simulink model "nuclearReactor"  (R2014b)
settings: Solver=ode1  StartTime=0.0  StopTime=100  FixedStep=0.0001  MaxStep=0.0001  RelTol=1e-3
(part 1 of 4)
settings Model: Creator=sand080  LastModifiedBy=nall426
settings DataIOCC: LimitDataPoints=off
settings RTWCC: CustomInitializer=gettimeofday(&t0, 0);
settings RTWCC: CustomSourceCode=|
  | int gettimeofday(struct timeval * tp, struct timezone * tzp)
  | {
  |     // Note: some broken versions only have 8 trailing zero's, the correct epoch has 9 trailing zero's
  |     static const uint64_t EPOCH = ((uint64_t) 116444736000000000ULL);
  | 
  |     SYSTEMTIME  system_time;
  |     FILETIME    file_time;
  |     uint64_t    time;
  | 
  | 	GetSystemTime( &system_time );
  |     SystemTimeToFileTime( &system_time, &file_time );
  |     time =  ((uint64_t)file_time.dwLowDateTime )      ;
  |     time += ((uint64_t)file_time.dwHighDateTime) << 32;
  | 
  |     tp->tv_sec  = (long) ((time - EPOCH) / 10000000L);
  |     tp->tv_usec = (long) (system_time.wMilliseconds * 1000);
  |     return 0;
  | }
  | 
  | struct timeval t0, t1;
settings RTWCC: CustomHeaderCode=|
  | #include <stdint.h> // portable: uint64_t   MSVC: __int64
  | #include <Windows.h>
settings RTWCC: CustomTerminator=|
  | gettimeofday(&t1, 0);
  | 
  | long elapsed = (t1.tv_sec-t0.tv_sec)*1000000 + t1.tv_usec-t0.tv_usec;
  | printf("Time taken: %ld microseconds (%.3f seconds)\n", elapsed, (elapsed / 1000000.0));

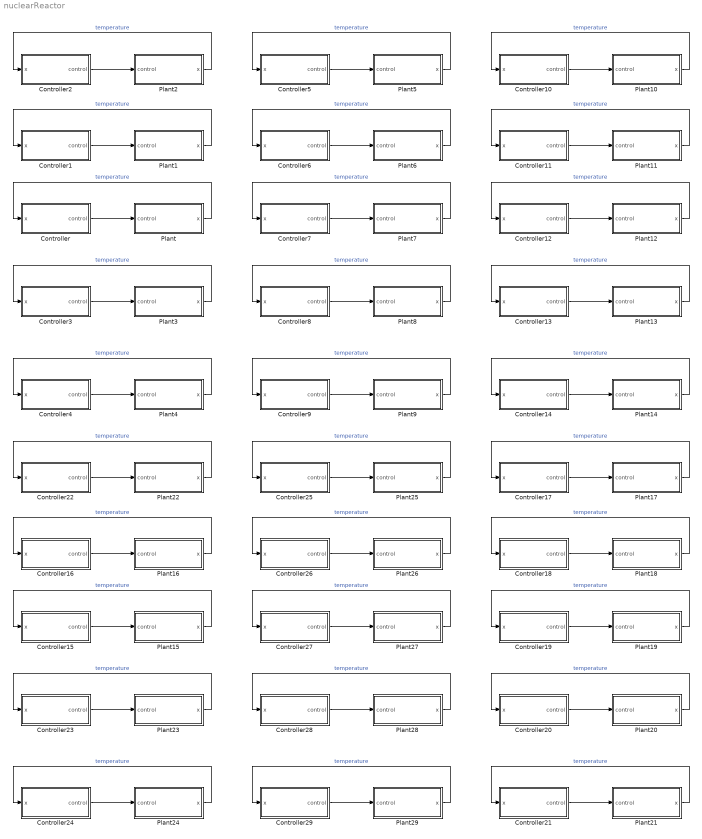
== system nuclearReactor ==
  Controller : Subsystem
  Controller1 : Subsystem
  Controller10 : Subsystem
  Controller11 : Subsystem
  Controller12 : Subsystem
  Controller13 : Subsystem
  Controller14 : Subsystem
  Controller15 : Subsystem
  Controller16 : Subsystem
  Controller17 : Subsystem
  Controller18 : Subsystem
  Controller19 : Subsystem
  Controller2 : Subsystem
  Controller20 : Subsystem
  Controller21 : Subsystem
  Controller22 : Subsystem
  Controller23 : Subsystem
  Controller24 : Subsystem
  Controller25 : Subsystem
  Controller26 : Subsystem
  Controller27 : Subsystem
  Controller28 : Subsystem
  Controller29 : Subsystem
  Controller3 : Subsystem
  Controller4 : Subsystem
  Controller5 : Subsystem
  Controller6 : Subsystem
  Controller7 : Subsystem
  Controller8 : Subsystem
  Controller9 : Subsystem
  Plant : Subsystem
  Plant1 : Subsystem
  Plant10 : Subsystem
  Plant11 : Subsystem
  Plant12 : Subsystem
  Plant13 : Subsystem
  Plant14 : Subsystem
  Plant15 : Subsystem
  Plant16 : Subsystem
  Plant17 : Subsystem
  Plant18 : Subsystem
  Plant19 : Subsystem
  Plant2 : Subsystem
  Plant20 : Subsystem
  Plant21 : Subsystem
  Plant22 : Subsystem
  Plant23 : Subsystem
  Plant24 : Subsystem
  Plant25 : Subsystem
  Plant26 : Subsystem
  Plant27 : Subsystem
  Plant28 : Subsystem
  Plant29 : Subsystem
  Plant3 : Subsystem
  Plant4 : Subsystem
  Plant5 : Subsystem
  Plant6 : Subsystem
  Plant7 : Subsystem
  Plant8 : Subsystem
  Plant9 : Subsystem
  wires:
  Controller/1(control) -> Plant/1(control)
  Plant/1(x) -> Controller/1(x)  "temperature"
  Controller1/1(control) -> Plant1/1(control)
  Plant1/1(x) -> Controller1/1(x)  "temperature"
  Controller2/1(control) -> Plant2/1(control)
  Plant2/1(x) -> Controller2/1(x)  "temperature"
  Controller3/1(control) -> Plant3/1(control)
  Plant3/1(x) -> Controller3/1(x)  "temperature"
  Controller4/1(control) -> Plant4/1(control)
  Plant4/1(x) -> Controller4/1(x)  "temperature"
  Controller5/1(control) -> Plant5/1(control)
  Plant5/1(x) -> Controller5/1(x)  "temperature"
  Controller6/1(control) -> Plant6/1(control)
  Plant6/1(x) -> Controller6/1(x)  "temperature"
  Controller7/1(control) -> Plant7/1(control)
  Plant7/1(x) -> Controller7/1(x)  "temperature"
  Controller8/1(control) -> Plant8/1(control)
  Plant8/1(x) -> Controller8/1(x)  "temperature"
  Controller9/1(control) -> Plant9/1(control)
  Plant9/1(x) -> Controller9/1(x)  "temperature"
  Controller10/1(control) -> Plant10/1(control)
  Plant10/1(x) -> Controller10/1(x)  "temperature"
  Controller11/1(control) -> Plant11/1(control)
  Plant11/1(x) -> Controller11/1(x)  "temperature"
  Controller12/1(control) -> Plant12/1(control)
  Plant12/1(x) -> Controller12/1(x)  "temperature"
  Controller13/1(control) -> Plant13/1(control)
  Plant13/1(x) -> Controller13/1(x)  "temperature"
  Controller14/1(control) -> Plant14/1(control)
  Plant14/1(x) -> Controller14/1(x)  "temperature"
  Controller15/1(control) -> Plant15/1(control)
  Plant15/1(x) -> Controller15/1(x)  "temperature"
  Controller16/1(control) -> Plant16/1(control)
  Plant16/1(x) -> Controller16/1(x)  "temperature"
  Controller22/1(control) -> Plant22/1(control)
  Plant22/1(x) -> Controller22/1(x)  "temperature"
  Controller23/1(control) -> Plant23/1(control)
  Plant23/1(x) -> Controller23/1(x)  "temperature"
  Controller24/1(control) -> Plant24/1(control)
  Plant24/1(x) -> Controller24/1(x)  "temperature"
  Controller25/1(control) -> Plant25/1(control)
  Plant25/1(x) -> Controller25/1(x)  "temperature"
  Controller26/1(control) -> Plant26/1(control)
  Plant26/1(x) -> Controller26/1(x)  "temperature"
  Controller27/1(control) -> Plant27/1(control)
  Plant27/1(x) -> Controller27/1(x)  "temperature"
  Controller28/1(control) -> Plant28/1(control)
  Plant28/1(x) -> Controller28/1(x)  "temperature"
  Controller29/1(control) -> Plant29/1(control)
  Plant29/1(x) -> Controller29/1(x)  "temperature"
  Controller17/1(control) -> Plant17/1(control)
  Plant17/1(x) -> Controller17/1(x)  "temperature"
  Controller18/1(control) -> Plant18/1(control)
  Plant18/1(x) -> Controller18/1(x)  "temperature"
  Controller19/1(control) -> Plant19/1(control)
  Plant19/1(x) -> Controller19/1(x)  "temperature"
  Controller20/1(control) -> Plant20/1(control)
  Plant20/1(x) -> Controller20/1(x)  "temperature"
  Controller21/1(control) -> Plant21/1(control)
  Plant21/1(x) -> Controller21/1(x)  "temperature"

== system nuclearReactor/Controller ==
  x : Inport
  INIT y1 : Constant  Value=0
  INIT y2 : Constant  Value=0
  Integrator t1 : DiscreteIntegrator  ExternalReset=either  InitialConditionSource=external  InitialCondition=510  InitialConditionSetting=State (most efficient)  SampleTime=-1
  Integrator t2 : DiscreteIntegrator  ExternalReset=either  InitialConditionSource=external  InitialCondition=510  InitialConditionSetting=State (most efficient)  SampleTime=-1
  MATLAB Function : MATLAB Function  Priority=1  TreatAsAtomicUnit=on
  Scope : Scope  NumInputPorts=8
      settings: TickLabels=on  ShowLegends=on  YMin=0~0~0~0~0~0~0~0  YMax=1~1~1~1~1~1~1~1
  con1 : Constant
  con2 : Constant
  q : Memory  LinearizeMemory=on
  reset1 : Memory  LinearizeMemory=on
  reset2 : Memory  LinearizeMemory=on
  control : Outport
  wires:
  MATLAB Function/4(control) -> Scope/1, control/1  "control"
  INIT y1/1 -> Integrator t1/3
  INIT y2/1 -> Integrator t2/3
  con1/1 -> Integrator t1/1
  MATLAB Function/1(qNext) -> q/1  "q_before"
  q/1 -> MATLAB Function/1(q)  "q_after"
  MATLAB Function/2(r1) -> reset1/1
  reset1/1 -> Integrator t1/2  "reset_after"
  x/1 -> Scope/8, MATLAB Function/2(x)
  con2/1 -> Integrator t2/1
  Integrator t1/1 -> MATLAB Function/3(y1), Scope/2  "integrator t1"
  Integrator t2/1 -> MATLAB Function/4(y2), Scope/3  "integrator t2"
  reset2/1 -> Integrator t2/2
  MATLAB Function/3(r2) -> reset2/1

== system nuclearReactor/Controller1 ==
  x : Inport
  INIT y1 : Constant  Value=0
  INIT y2 : Constant  Value=0
  Integrator t1 : DiscreteIntegrator  ExternalReset=either  InitialConditionSource=external  InitialCondition=510  InitialConditionSetting=State (most efficient)  SampleTime=-1
  Integrator t2 : DiscreteIntegrator  ExternalReset=either  InitialConditionSource=external  InitialCondition=510  InitialConditionSetting=State (most efficient)  SampleTime=-1
  MATLAB Function : MATLAB Function  Priority=1  TreatAsAtomicUnit=on
  Scope : Scope  NumInputPorts=8
      settings: TickLabels=on  ShowLegends=on  YMin=0~0~0~0~0~0~0~0  YMax=1~1~1~1~1~1~1~1
  con1 : Constant
  con2 : Constant
  q : Memory  LinearizeMemory=on
  reset1 : Memory  LinearizeMemory=on
  reset2 : Memory  LinearizeMemory=on
  control : Outport
  wires:
  MATLAB Function/4(control) -> Scope/1, control/1  "control"
  INIT y1/1 -> Integrator t1/3
  INIT y2/1 -> Integrator t2/3
  con1/1 -> Integrator t1/1
  MATLAB Function/1(qNext) -> q/1  "q_before"
  q/1 -> MATLAB Function/1(q)  "q_after"
  MATLAB Function/2(r1) -> reset1/1
  reset1/1 -> Integrator t1/2  "reset_after"
  x/1 -> Scope/8, MATLAB Function/2(x)
  con2/1 -> Integrator t2/1
  Integrator t1/1 -> MATLAB Function/3(y1), Scope/2  "integrator t1"
  Integrator t2/1 -> MATLAB Function/4(y2), Scope/3  "integrator t2"
  reset2/1 -> Integrator t2/2
  MATLAB Function/3(r2) -> reset2/1

== system nuclearReactor/Controller10 ==
  x : Inport
  INIT y1 : Constant  Value=0
  INIT y2 : Constant  Value=0
  Integrator t1 : DiscreteIntegrator  ExternalReset=either  InitialConditionSource=external  InitialCondition=510  InitialConditionSetting=State (most efficient)  SampleTime=-1
  Integrator t2 : DiscreteIntegrator  ExternalReset=either  InitialConditionSource=external  InitialCondition=510  InitialConditionSetting=State (most efficient)  SampleTime=-1
  MATLAB Function : MATLAB Function  Priority=1  TreatAsAtomicUnit=on
  Scope : Scope  NumInputPorts=8
      settings: TickLabels=on  ShowLegends=on  YMin=0~0~0~0~0~0~0~0  YMax=1~1~1~1~1~1~1~1
  con1 : Constant
  con2 : Constant
  q : Memory  LinearizeMemory=on
  reset1 : Memory  LinearizeMemory=on
  reset2 : Memory  LinearizeMemory=on
  control : Outport
  wires:
  MATLAB Function/4(control) -> Scope/1, control/1  "control"
  INIT y1/1 -> Integrator t1/3
  INIT y2/1 -> Integrator t2/3
  con1/1 -> Integrator t1/1
  MATLAB Function/1(qNext) -> q/1  "q_before"
  q/1 -> MATLAB Function/1(q)  "q_after"
  MATLAB Function/2(r1) -> reset1/1
  reset1/1 -> Integrator t1/2  "reset_after"
  x/1 -> Scope/8, MATLAB Function/2(x)
  con2/1 -> Integrator t2/1
  Integrator t1/1 -> MATLAB Function/3(y1), Scope/2  "integrator t1"
  Integrator t2/1 -> MATLAB Function/4(y2), Scope/3  "integrator t2"
  reset2/1 -> Integrator t2/2
  MATLAB Function/3(r2) -> reset2/1

== system nuclearReactor/Controller11 ==
  x : Inport
  INIT y1 : Constant  Value=0
  INIT y2 : Constant  Value=0
  Integrator t1 : DiscreteIntegrator  ExternalReset=either  InitialConditionSource=external  InitialCondition=510  InitialConditionSetting=State (most efficient)  SampleTime=-1
  Integrator t2 : DiscreteIntegrator  ExternalReset=either  InitialConditionSource=external  InitialCondition=510  InitialConditionSetting=State (most efficient)  SampleTime=-1
  MATLAB Function : MATLAB Function  Priority=1  TreatAsAtomicUnit=on
  Scope : Scope  NumInputPorts=8
      settings: TickLabels=on  ShowLegends=on  YMin=0~0~0~0~0~0~0~0  YMax=1~1~1~1~1~1~1~1
  con1 : Constant
  con2 : Constant
  q : Memory  LinearizeMemory=on
  reset1 : Memory  LinearizeMemory=on
  reset2 : Memory  LinearizeMemory=on
  control : Outport
  wires:
  MATLAB Function/4(control) -> Scope/1, control/1  "control"
  INIT y1/1 -> Integrator t1/3
  INIT y2/1 -> Integrator t2/3
  con1/1 -> Integrator t1/1
  MATLAB Function/1(qNext) -> q/1  "q_before"
  q/1 -> MATLAB Function/1(q)  "q_after"
  MATLAB Function/2(r1) -> reset1/1
  reset1/1 -> Integrator t1/2  "reset_after"
  x/1 -> Scope/8, MATLAB Function/2(x)
  con2/1 -> Integrator t2/1
  Integrator t1/1 -> MATLAB Function/3(y1), Scope/2  "integrator t1"
  Integrator t2/1 -> MATLAB Function/4(y2), Scope/3  "integrator t2"
  reset2/1 -> Integrator t2/2
  MATLAB Function/3(r2) -> reset2/1

== system nuclearReactor/Controller12 ==
  x : Inport
  INIT y1 : Constant  Value=0
  INIT y2 : Constant  Value=0
  Integrator t1 : DiscreteIntegrator  ExternalReset=either  InitialConditionSource=external  InitialCondition=510  InitialConditionSetting=State (most efficient)  SampleTime=-1
  Integrator t2 : DiscreteIntegrator  ExternalReset=either  InitialConditionSource=external  InitialCondition=510  InitialConditionSetting=State (most efficient)  SampleTime=-1
  MATLAB Function : MATLAB Function  Priority=1  TreatAsAtomicUnit=on
  Scope : Scope  NumInputPorts=8
      settings: TickLabels=on  ShowLegends=on  YMin=0~0~0~0~0~0~0~0  YMax=1~1~1~1~1~1~1~1
  con1 : Constant
  con2 : Constant
  q : Memory  LinearizeMemory=on
  reset1 : Memory  LinearizeMemory=on
  reset2 : Memory  LinearizeMemory=on
  control : Outport
  wires:
  MATLAB Function/4(control) -> Scope/1, control/1  "control"
  INIT y1/1 -> Integrator t1/3
  INIT y2/1 -> Integrator t2/3
  con1/1 -> Integrator t1/1
  MATLAB Function/1(qNext) -> q/1  "q_before"
  q/1 -> MATLAB Function/1(q)  "q_after"
  MATLAB Function/2(r1) -> reset1/1
  reset1/1 -> Integrator t1/2  "reset_after"
  x/1 -> Scope/8, MATLAB Function/2(x)
  con2/1 -> Integrator t2/1
  Integrator t1/1 -> MATLAB Function/3(y1), Scope/2  "integrator t1"
  Integrator t2/1 -> MATLAB Function/4(y2), Scope/3  "integrator t2"
  reset2/1 -> Integrator t2/2
  MATLAB Function/3(r2) -> reset2/1

== system nuclearReactor/Controller13 ==
  x : Inport
  INIT y1 : Constant  Value=0
  INIT y2 : Constant  Value=0
  Integrator t1 : DiscreteIntegrator  ExternalReset=either  InitialConditionSource=external  InitialCondition=510  InitialConditionSetting=State (most efficient)  SampleTime=-1
  Integrator t2 : DiscreteIntegrator  ExternalReset=either  InitialConditionSource=external  InitialCondition=510  InitialConditionSetting=State (most efficient)  SampleTime=-1
  MATLAB Function : MATLAB Function  Priority=1  TreatAsAtomicUnit=on
  Scope : Scope  NumInputPorts=8
      settings: TickLabels=on  ShowLegends=on  YMin=0~0~0~0~0~0~0~0  YMax=1~1~1~1~1~1~1~1
  con1 : Constant
  con2 : Constant
  q : Memory  LinearizeMemory=on
  reset1 : Memory  LinearizeMemory=on
  reset2 : Memory  LinearizeMemory=on
  control : Outport
  wires:
  MATLAB Function/4(control) -> Scope/1, control/1  "control"
  INIT y1/1 -> Integrator t1/3
  INIT y2/1 -> Integrator t2/3
  con1/1 -> Integrator t1/1
  MATLAB Function/1(qNext) -> q/1  "q_before"
  q/1 -> MATLAB Function/1(q)  "q_after"
  MATLAB Function/2(r1) -> reset1/1
  reset1/1 -> Integrator t1/2  "reset_after"
  x/1 -> Scope/8, MATLAB Function/2(x)
  con2/1 -> Integrator t2/1
  Integrator t1/1 -> MATLAB Function/3(y1), Scope/2  "integrator t1"
  Integrator t2/1 -> MATLAB Function/4(y2), Scope/3  "integrator t2"
  reset2/1 -> Integrator t2/2
  MATLAB Function/3(r2) -> reset2/1

== system nuclearReactor/Controller14 ==
  x : Inport
  INIT y1 : Constant  Value=0
  INIT y2 : Constant  Value=0
  Integrator t1 : DiscreteIntegrator  ExternalReset=either  InitialConditionSource=external  InitialCondition=510  InitialConditionSetting=State (most efficient)  SampleTime=-1
  Integrator t2 : DiscreteIntegrator  ExternalReset=either  InitialConditionSource=external  InitialCondition=510  InitialConditionSetting=State (most efficient)  SampleTime=-1
  MATLAB Function : MATLAB Function  Priority=1  TreatAsAtomicUnit=on
  Scope : Scope  NumInputPorts=8
      settings: TickLabels=on  ShowLegends=on  YMin=0~0~0~0~0~0~0~0  YMax=1~1~1~1~1~1~1~1
  con1 : Constant
  con2 : Constant
  q : Memory  LinearizeMemory=on
  reset1 : Memory  LinearizeMemory=on
  reset2 : Memory  LinearizeMemory=on
  control : Outport
  wires:
  MATLAB Function/4(control) -> Scope/1, control/1  "control"
  INIT y1/1 -> Integrator t1/3
  INIT y2/1 -> Integrator t2/3
  con1/1 -> Integrator t1/1
  MATLAB Function/1(qNext) -> q/1  "q_before"
  q/1 -> MATLAB Function/1(q)  "q_after"
  MATLAB Function/2(r1) -> reset1/1
  reset1/1 -> Integrator t1/2  "reset_after"
  x/1 -> Scope/8, MATLAB Function/2(x)
  con2/1 -> Integrator t2/1
  Integrator t1/1 -> MATLAB Function/3(y1), Scope/2  "integrator t1"
  Integrator t2/1 -> MATLAB Function/4(y2), Scope/3  "integrator t2"
  reset2/1 -> Integrator t2/2
  MATLAB Function/3(r2) -> reset2/1

== system nuclearReactor/Controller15 ==
  x : Inport
  INIT y1 : Constant  Value=0
  INIT y2 : Constant  Value=0
  Integrator t1 : DiscreteIntegrator  ExternalReset=either  InitialConditionSource=external  InitialCondition=510  InitialConditionSetting=State (most efficient)  SampleTime=-1
  Integrator t2 : DiscreteIntegrator  ExternalReset=either  InitialConditionSource=external  InitialCondition=510  InitialConditionSetting=State (most efficient)  SampleTime=-1
  MATLAB Function : MATLAB Function  Priority=1  TreatAsAtomicUnit=on
  Scope : Scope  NumInputPorts=8
      settings: TickLabels=on  ShowLegends=on  YMin=0~0~0~0~0~0~0~0  YMax=1~1~1~1~1~1~1~1
  con1 : Constant
  con2 : Constant
  q : Memory  LinearizeMemory=on
  reset1 : Memory  LinearizeMemory=on
  reset2 : Memory  LinearizeMemory=on
  control : Outport
  wires:
  MATLAB Function/4(control) -> Scope/1, control/1  "control"
  INIT y1/1 -> Integrator t1/3
  INIT y2/1 -> Integrator t2/3
  con1/1 -> Integrator t1/1
  MATLAB Function/1(qNext) -> q/1  "q_before"
  q/1 -> MATLAB Function/1(q)  "q_after"
  MATLAB Function/2(r1) -> reset1/1
  reset1/1 -> Integrator t1/2  "reset_after"
  x/1 -> Scope/8, MATLAB Function/2(x)
  con2/1 -> Integrator t2/1
  Integrator t1/1 -> MATLAB Function/3(y1), Scope/2  "integrator t1"
  Integrator t2/1 -> MATLAB Function/4(y2), Scope/3  "integrator t2"
  reset2/1 -> Integrator t2/2
  MATLAB Function/3(r2) -> reset2/1

== system nuclearReactor/Controller16 ==
  x : Inport
  INIT y1 : Constant  Value=0
  INIT y2 : Constant  Value=0
  Integrator t1 : DiscreteIntegrator  ExternalReset=either  InitialConditionSource=external  InitialCondition=510  InitialConditionSetting=State (most efficient)  SampleTime=-1
  Integrator t2 : DiscreteIntegrator  ExternalReset=either  InitialConditionSource=external  InitialCondition=510  InitialConditionSetting=State (most efficient)  SampleTime=-1
  MATLAB Function : MATLAB Function  Priority=1  TreatAsAtomicUnit=on
  Scope : Scope  NumInputPorts=8
      settings: TickLabels=on  ShowLegends=on  YMin=0~0~0~0~0~0~0~0  YMax=1~1~1~1~1~1~1~1
  con1 : Constant
  con2 : Constant
  q : Memory  LinearizeMemory=on
  reset1 : Memory  LinearizeMemory=on
  reset2 : Memory  LinearizeMemory=on
  control : Outport
  wires:
  MATLAB Function/4(control) -> Scope/1, control/1  "control"
  INIT y1/1 -> Integrator t1/3
  INIT y2/1 -> Integrator t2/3
  con1/1 -> Integrator t1/1
  MATLAB Function/1(qNext) -> q/1  "q_before"
  q/1 -> MATLAB Function/1(q)  "q_after"
  MATLAB Function/2(r1) -> reset1/1
  reset1/1 -> Integrator t1/2  "reset_after"
  x/1 -> Scope/8, MATLAB Function/2(x)
  con2/1 -> Integrator t2/1
  Integrator t1/1 -> MATLAB Function/3(y1), Scope/2  "integrator t1"
  Integrator t2/1 -> MATLAB Function/4(y2), Scope/3  "integrator t2"
  reset2/1 -> Integrator t2/2
  MATLAB Function/3(r2) -> reset2/1

== system nuclearReactor/Controller17 ==
  x : Inport
  INIT y1 : Constant  Value=0
  INIT y2 : Constant  Value=0
  Integrator t1 : DiscreteIntegrator  ExternalReset=either  InitialConditionSource=external  InitialCondition=510  InitialConditionSetting=State (most efficient)  SampleTime=-1
  Integrator t2 : DiscreteIntegrator  ExternalReset=either  InitialConditionSource=external  InitialCondition=510  InitialConditionSetting=State (most efficient)  SampleTime=-1
  MATLAB Function : MATLAB Function  Priority=1  TreatAsAtomicUnit=on
  Scope : Scope  NumInputPorts=8
      settings: TickLabels=on  ShowLegends=on  YMin=0~0~0~0~0~0~0~0  YMax=1~1~1~1~1~1~1~1
  con1 : Constant
  con2 : Constant
  q : Memory  LinearizeMemory=on
  reset1 : Memory  LinearizeMemory=on
  reset2 : Memory  LinearizeMemory=on
  control : Outport
  wires:
  MATLAB Function/4(control) -> Scope/1, control/1  "control"
  INIT y1/1 -> Integrator t1/3
  INIT y2/1 -> Integrator t2/3
  con1/1 -> Integrator t1/1
  MATLAB Function/1(qNext) -> q/1  "q_before"
  q/1 -> MATLAB Function/1(q)  "q_after"
  MATLAB Function/2(r1) -> reset1/1
  reset1/1 -> Integrator t1/2  "reset_after"
  x/1 -> Scope/8, MATLAB Function/2(x)
  con2/1 -> Integrator t2/1
  Integrator t1/1 -> MATLAB Function/3(y1), Scope/2  "integrator t1"
  Integrator t2/1 -> MATLAB Function/4(y2), Scope/3  "integrator t2"
  reset2/1 -> Integrator t2/2
  MATLAB Function/3(r2) -> reset2/1

== system nuclearReactor/Controller18 ==
  x : Inport
  INIT y1 : Constant  Value=0
  INIT y2 : Constant  Value=0
  Integrator t1 : DiscreteIntegrator  ExternalReset=either  InitialConditionSource=external  InitialCondition=510  InitialConditionSetting=State (most efficient)  SampleTime=-1
  Integrator t2 : DiscreteIntegrator  ExternalReset=either  InitialConditionSource=external  InitialCondition=510  InitialConditionSetting=State (most efficient)  SampleTime=-1
  MATLAB Function : MATLAB Function  Priority=1  TreatAsAtomicUnit=on
  Scope : Scope  NumInputPorts=8
      settings: TickLabels=on  ShowLegends=on  YMin=0~0~0~0~0~0~0~0  YMax=1~1~1~1~1~1~1~1
  con1 : Constant
  con2 : Constant
  q : Memory  LinearizeMemory=on
  reset1 : Memory  LinearizeMemory=on
  reset2 : Memory  LinearizeMemory=on
  control : Outport
  wires:
  MATLAB Function/4(control) -> Scope/1, control/1  "control"
  INIT y1/1 -> Integrator t1/3
  INIT y2/1 -> Integrator t2/3
  con1/1 -> Integrator t1/1
  MATLAB Function/1(qNext) -> q/1  "q_before"
  q/1 -> MATLAB Function/1(q)  "q_after"
  MATLAB Function/2(r1) -> reset1/1
  reset1/1 -> Integrator t1/2  "reset_after"
  x/1 -> Scope/8, MATLAB Function/2(x)
  con2/1 -> Integrator t2/1
  Integrator t1/1 -> MATLAB Function/3(y1), Scope/2  "integrator t1"
  Integrator t2/1 -> MATLAB Function/4(y2), Scope/3  "integrator t2"
  reset2/1 -> Integrator t2/2
  MATLAB Function/3(r2) -> reset2/1

== system nuclearReactor/Controller19 ==
  x : Inport
  INIT y1 : Constant  Value=0
  INIT y2 : Constant  Value=0
  Integrator t1 : DiscreteIntegrator  ExternalReset=either  InitialConditionSource=external  InitialCondition=510  InitialConditionSetting=State (most efficient)  SampleTime=-1
  Integrator t2 : DiscreteIntegrator  ExternalReset=either  InitialConditionSource=external  InitialCondition=510  InitialConditionSetting=State (most efficient)  SampleTime=-1
  MATLAB Function : MATLAB Function  Priority=1  TreatAsAtomicUnit=on
  Scope : Scope  NumInputPorts=8
      settings: TickLabels=on  ShowLegends=on  YMin=0~0~0~0~0~0~0~0  YMax=1~1~1~1~1~1~1~1
  con1 : Constant
  con2 : Constant
  q : Memory  LinearizeMemory=on
  reset1 : Memory  LinearizeMemory=on
  reset2 : Memory  LinearizeMemory=on
  control : Outport
  wires:
  MATLAB Function/4(control) -> Scope/1, control/1  "control"
  INIT y1/1 -> Integrator t1/3
  INIT y2/1 -> Integrator t2/3
  con1/1 -> Integrator t1/1
  MATLAB Function/1(qNext) -> q/1  "q_before"
  q/1 -> MATLAB Function/1(q)  "q_after"
  MATLAB Function/2(r1) -> reset1/1
  reset1/1 -> Integrator t1/2  "reset_after"
  x/1 -> Scope/8, MATLAB Function/2(x)
  con2/1 -> Integrator t2/1
  Integrator t1/1 -> MATLAB Function/3(y1), Scope/2  "integrator t1"
  Integrator t2/1 -> MATLAB Function/4(y2), Scope/3  "integrator t2"
  reset2/1 -> Integrator t2/2
  MATLAB Function/3(r2) -> reset2/1

== system nuclearReactor/Controller2 ==
  x : Inport
  INIT y1 : Constant  Value=0
  INIT y2 : Constant  Value=0
  Integrator t1 : DiscreteIntegrator  ExternalReset=either  InitialConditionSource=external  InitialCondition=510  InitialConditionSetting=State (most efficient)  SampleTime=-1
  Integrator t2 : DiscreteIntegrator  ExternalReset=either  InitialConditionSource=external  InitialCondition=510  InitialConditionSetting=State (most efficient)  SampleTime=-1
  MATLAB Function : MATLAB Function  Priority=1  TreatAsAtomicUnit=on
  Scope : Scope  NumInputPorts=8
      settings: TickLabels=on  ShowLegends=on  YMin=0~0~0~0~0~0~0~0  YMax=1~1~1~1~1~1~1~1
  con1 : Constant
  con2 : Constant
  q : Memory  LinearizeMemory=on
  reset1 : Memory  LinearizeMemory=on
  reset2 : Memory  LinearizeMemory=on
  control : Outport
  wires:
  MATLAB Function/4(control) -> Scope/1, control/1  "control"
  INIT y1/1 -> Integrator t1/3
  INIT y2/1 -> Integrator t2/3
  con1/1 -> Integrator t1/1
  MATLAB Function/1(qNext) -> q/1  "q_before"
  q/1 -> MATLAB Function/1(q)  "q_after"
  MATLAB Function/2(r1) -> reset1/1
  reset1/1 -> Integrator t1/2  "reset_after"
  x/1 -> Scope/8, MATLAB Function/2(x)
  con2/1 -> Integrator t2/1
  Integrator t1/1 -> MATLAB Function/3(y1), Scope/2  "integrator t1"
  Integrator t2/1 -> MATLAB Function/4(y2), Scope/3  "integrator t2"
  reset2/1 -> Integrator t2/2
  MATLAB Function/3(r2) -> reset2/1

== system nuclearReactor/Controller20 ==
  x : Inport
  INIT y1 : Constant  Value=0
  INIT y2 : Constant  Value=0
  Integrator t1 : DiscreteIntegrator  ExternalReset=either  InitialConditionSource=external  InitialCondition=510  InitialConditionSetting=State (most efficient)  SampleTime=-1
  Integrator t2 : DiscreteIntegrator  ExternalReset=either  InitialConditionSource=external  InitialCondition=510  InitialConditionSetting=State (most efficient)  SampleTime=-1
  MATLAB Function : MATLAB Function  Priority=1  TreatAsAtomicUnit=on
  Scope : Scope  NumInputPorts=8
      settings: TickLabels=on  ShowLegends=on  YMin=0~0~0~0~0~0~0~0  YMax=1~1~1~1~1~1~1~1
  con1 : Constant
  con2 : Constant
  q : Memory  LinearizeMemory=on
  reset1 : Memory  LinearizeMemory=on
  reset2 : Memory  LinearizeMemory=on
  control : Outport
  wires:
  MATLAB Function/4(control) -> Scope/1, control/1  "control"
  INIT y1/1 -> Integrator t1/3
  INIT y2/1 -> Integrator t2/3
  con1/1 -> Integrator t1/1
  MATLAB Function/1(qNext) -> q/1  "q_before"
  q/1 -> MATLAB Function/1(q)  "q_after"
  MATLAB Function/2(r1) -> reset1/1
  reset1/1 -> Integrator t1/2  "reset_after"
  x/1 -> Scope/8, MATLAB Function/2(x)
  con2/1 -> Integrator t2/1
  Integrator t1/1 -> MATLAB Function/3(y1), Scope/2  "integrator t1"
  Integrator t2/1 -> MATLAB Function/4(y2), Scope/3  "integrator t2"
  reset2/1 -> Integrator t2/2
  MATLAB Function/3(r2) -> reset2/1

== system nuclearReactor/Controller21 ==
  x : Inport
  INIT y1 : Constant  Value=0
  INIT y2 : Constant  Value=0
  Integrator t1 : DiscreteIntegrator  ExternalReset=either  InitialConditionSource=external  InitialCondition=510  InitialConditionSetting=State (most efficient)  SampleTime=-1
  Integrator t2 : DiscreteIntegrator  ExternalReset=either  InitialConditionSource=external  InitialCondition=510  InitialConditionSetting=State (most efficient)  SampleTime=-1
  MATLAB Function : MATLAB Function  Priority=1  TreatAsAtomicUnit=on
  Scope : Scope  NumInputPorts=8
      settings: TickLabels=on  ShowLegends=on  YMin=0~0~0~0~0~0~0~0  YMax=1~1~1~1~1~1~1~1
  con1 : Constant
  con2 : Constant
  q : Memory  LinearizeMemory=on
  reset1 : Memory  LinearizeMemory=on
  reset2 : Memory  LinearizeMemory=on
  control : Outport
  wires:
  MATLAB Function/4(control) -> Scope/1, control/1  "control"
  INIT y1/1 -> Integrator t1/3
  INIT y2/1 -> Integrator t2/3
  con1/1 -> Integrator t1/1
  MATLAB Function/1(qNext) -> q/1  "q_before"
  q/1 -> MATLAB Function/1(q)  "q_after"
  MATLAB Function/2(r1) -> reset1/1
  reset1/1 -> Integrator t1/2  "reset_after"
  x/1 -> Scope/8, MATLAB Function/2(x)
  con2/1 -> Integrator t2/1
  Integrator t1/1 -> MATLAB Function/3(y1), Scope/2  "integrator t1"
  Integrator t2/1 -> MATLAB Function/4(y2), Scope/3  "integrator t2"
  reset2/1 -> Integrator t2/2
  MATLAB Function/3(r2) -> reset2/1

== system nuclearReactor/Controller22 ==
  x : Inport
  INIT y1 : Constant  Value=0
  INIT y2 : Constant  Value=0
  Integrator t1 : DiscreteIntegrator  ExternalReset=either  InitialConditionSource=external  InitialCondition=510  InitialConditionSetting=State (most efficient)  SampleTime=-1
  Integrator t2 : DiscreteIntegrator  ExternalReset=either  InitialConditionSource=external  InitialCondition=510  InitialConditionSetting=State (most efficient)  SampleTime=-1
  MATLAB Function : MATLAB Function  Priority=1  TreatAsAtomicUnit=on
  Scope : Scope  NumInputPorts=8
      settings: TickLabels=on  ShowLegends=on  YMin=0~0~0~0~0~0~0~0  YMax=1~1~1~1~1~1~1~1
  con1 : Constant
  con2 : Constant
  q : Memory  LinearizeMemory=on
  reset1 : Memory  LinearizeMemory=on
  reset2 : Memory  LinearizeMemory=on
  control : Outport
  wires:
  MATLAB Function/4(control) -> Scope/1, control/1  "control"
  INIT y1/1 -> Integrator t1/3
  INIT y2/1 -> Integrator t2/3
  con1/1 -> Integrator t1/1
  MATLAB Function/1(qNext) -> q/1  "q_before"
  q/1 -> MATLAB Function/1(q)  "q_after"
  MATLAB Function/2(r1) -> reset1/1
  reset1/1 -> Integrator t1/2  "reset_after"
  x/1 -> Scope/8, MATLAB Function/2(x)
  con2/1 -> Integrator t2/1
  Integrator t1/1 -> MATLAB Function/3(y1), Scope/2  "integrator t1"
  Integrator t2/1 -> MATLAB Function/4(y2), Scope/3  "integrator t2"
  reset2/1 -> Integrator t2/2
  MATLAB Function/3(r2) -> reset2/1

== system nuclearReactor/Controller23 ==
  x : Inport
  INIT y1 : Constant  Value=0
  INIT y2 : Constant  Value=0
  Integrator t1 : DiscreteIntegrator  ExternalReset=either  InitialConditionSource=external  InitialCondition=510  InitialConditionSetting=State (most efficient)  SampleTime=-1
  Integrator t2 : DiscreteIntegrator  ExternalReset=either  InitialConditionSource=external  InitialCondition=510  InitialConditionSetting=State (most efficient)  SampleTime=-1
  MATLAB Function : MATLAB Function  Priority=1  TreatAsAtomicUnit=on
  Scope : Scope  NumInputPorts=8
      settings: TickLabels=on  ShowLegends=on  YMin=0~0~0~0~0~0~0~0  YMax=1~1~1~1~1~1~1~1
  con1 : Constant
  con2 : Constant
  q : Memory  LinearizeMemory=on
  reset1 : Memory  LinearizeMemory=on
  reset2 : Memory  LinearizeMemory=on
  control : Outport
  wires:
  MATLAB Function/4(control) -> Scope/1, control/1  "control"
  INIT y1/1 -> Integrator t1/3
  INIT y2/1 -> Integrator t2/3
  con1/1 -> Integrator t1/1
  MATLAB Function/1(qNext) -> q/1  "q_before"
  q/1 -> MATLAB Function/1(q)  "q_after"
  MATLAB Function/2(r1) -> reset1/1
  reset1/1 -> Integrator t1/2  "reset_after"
  x/1 -> Scope/8, MATLAB Function/2(x)
  con2/1 -> Integrator t2/1
  Integrator t1/1 -> MATLAB Function/3(y1), Scope/2  "integrator t1"
  Integrator t2/1 -> MATLAB Function/4(y2), Scope/3  "integrator t2"
  reset2/1 -> Integrator t2/2
  MATLAB Function/3(r2) -> reset2/1

== system nuclearReactor/Controller24 ==
  x : Inport
  INIT y1 : Constant  Value=0
  INIT y2 : Constant  Value=0
  Integrator t1 : DiscreteIntegrator  ExternalReset=either  InitialConditionSource=external  InitialCondition=510  InitialConditionSetting=State (most efficient)  SampleTime=-1
  Integrator t2 : DiscreteIntegrator  ExternalReset=either  InitialConditionSource=external  InitialCondition=510  InitialConditionSetting=State (most efficient)  SampleTime=-1
  MATLAB Function : MATLAB Function  Priority=1  TreatAsAtomicUnit=on
  Scope : Scope  NumInputPorts=8
      settings: TickLabels=on  ShowLegends=on  YMin=0~0~0~0~0~0~0~0  YMax=1~1~1~1~1~1~1~1
  con1 : Constant
  con2 : Constant
  q : Memory  LinearizeMemory=on
  reset1 : Memory  LinearizeMemory=on
  reset2 : Memory  LinearizeMemory=on
  control : Outport
  wires:
  MATLAB Function/4(control) -> Scope/1, control/1  "control"
  INIT y1/1 -> Integrator t1/3
  INIT y2/1 -> Integrator t2/3
  con1/1 -> Integrator t1/1
  MATLAB Function/1(qNext) -> q/1  "q_before"
  q/1 -> MATLAB Function/1(q)  "q_after"
  MATLAB Function/2(r1) -> reset1/1
  reset1/1 -> Integrator t1/2  "reset_after"
  x/1 -> Scope/8, MATLAB Function/2(x)
  con2/1 -> Integrator t2/1
  Integrator t1/1 -> MATLAB Function/3(y1), Scope/2  "integrator t1"
  Integrator t2/1 -> MATLAB Function/4(y2), Scope/3  "integrator t2"
  reset2/1 -> Integrator t2/2
  MATLAB Function/3(r2) -> reset2/1

== system nuclearReactor/Controller25 ==
  x : Inport
  INIT y1 : Constant  Value=0
  INIT y2 : Constant  Value=0
  Integrator t1 : DiscreteIntegrator  ExternalReset=either  InitialConditionSource=external  InitialCondition=510  InitialConditionSetting=State (most efficient)  SampleTime=-1
  Integrator t2 : DiscreteIntegrator  ExternalReset=either  InitialConditionSource=external  InitialCondition=510  InitialConditionSetting=State (most efficient)  SampleTime=-1
  MATLAB Function : MATLAB Function  Priority=1  TreatAsAtomicUnit=on
  Scope : Scope  NumInputPorts=8
      settings: TickLabels=on  ShowLegends=on  YMin=0~0~0~0~0~0~0~0  YMax=1~1~1~1~1~1~1~1
  con1 : Constant
  con2 : Constant
  q : Memory  LinearizeMemory=on
  reset1 : Memory  LinearizeMemory=on
  reset2 : Memory  LinearizeMemory=on
  control : Outport
  wires:
  MATLAB Function/4(control) -> Scope/1, control/1  "control"
  INIT y1/1 -> Integrator t1/3
  INIT y2/1 -> Integrator t2/3
  con1/1 -> Integrator t1/1
  MATLAB Function/1(qNext) -> q/1  "q_before"
  q/1 -> MATLAB Function/1(q)  "q_after"
  MATLAB Function/2(r1) -> reset1/1
  reset1/1 -> Integrator t1/2  "reset_after"
  x/1 -> Scope/8, MATLAB Function/2(x)
  con2/1 -> Integrator t2/1
  Integrator t1/1 -> MATLAB Function/3(y1), Scope/2  "integrator t1"
  Integrator t2/1 -> MATLAB Function/4(y2), Scope/3  "integrator t2"
  reset2/1 -> Integrator t2/2
  MATLAB Function/3(r2) -> reset2/1

== system nuclearReactor/Controller26 ==
  x : Inport
  INIT y1 : Constant  Value=0
  INIT y2 : Constant  Value=0
  Integrator t1 : DiscreteIntegrator  ExternalReset=either  InitialConditionSource=external  InitialCondition=510  InitialConditionSetting=State (most efficient)  SampleTime=-1
  Integrator t2 : DiscreteIntegrator  ExternalReset=either  InitialConditionSource=external  InitialCondition=510  InitialConditionSetting=State (most efficient)  SampleTime=-1
  MATLAB Function : MATLAB Function  Priority=1  TreatAsAtomicUnit=on
  Scope : Scope  NumInputPorts=8
      settings: TickLabels=on  ShowLegends=on  YMin=0~0~0~0~0~0~0~0  YMax=1~1~1~1~1~1~1~1
  con1 : Constant
  con2 : Constant
  q : Memory  LinearizeMemory=on
  reset1 : Memory  LinearizeMemory=on
  reset2 : Memory  LinearizeMemory=on
  control : Outport
  wires:
  MATLAB Function/4(control) -> Scope/1, control/1  "control"
  INIT y1/1 -> Integrator t1/3
  INIT y2/1 -> Integrator t2/3
  con1/1 -> Integrator t1/1
  MATLAB Function/1(qNext) -> q/1  "q_before"
  q/1 -> MATLAB Function/1(q)  "q_after"
  MATLAB Function/2(r1) -> reset1/1
  reset1/1 -> Integrator t1/2  "reset_after"
  x/1 -> Scope/8, MATLAB Function/2(x)
  con2/1 -> Integrator t2/1
  Integrator t1/1 -> MATLAB Function/3(y1), Scope/2  "integrator t1"
  Integrator t2/1 -> MATLAB Function/4(y2), Scope/3  "integrator t2"
  reset2/1 -> Integrator t2/2
  MATLAB Function/3(r2) -> reset2/1

== system nuclearReactor/Controller27 ==
  x : Inport
  INIT y1 : Constant  Value=0
  INIT y2 : Constant  Value=0
  Integrator t1 : DiscreteIntegrator  ExternalReset=either  InitialConditionSource=external  InitialCondition=510  InitialConditionSetting=State (most efficient)  SampleTime=-1
  Integrator t2 : DiscreteIntegrator  ExternalReset=either  InitialConditionSource=external  InitialCondition=510  InitialConditionSetting=State (most efficient)  SampleTime=-1
  MATLAB Function : MATLAB Function  Priority=1  TreatAsAtomicUnit=on
  Scope : Scope  NumInputPorts=8
      settings: TickLabels=on  ShowLegends=on  YMin=0~0~0~0~0~0~0~0  YMax=1~1~1~1~1~1~1~1
  con1 : Constant
  con2 : Constant
  q : Memory  LinearizeMemory=on
  reset1 : Memory  LinearizeMemory=on
  reset2 : Memory  LinearizeMemory=on
  control : Outport
  wires:
  MATLAB Function/4(control) -> Scope/1, control/1  "control"
  INIT y1/1 -> Integrator t1/3
  INIT y2/1 -> Integrator t2/3
  con1/1 -> Integrator t1/1
  MATLAB Function/1(qNext) -> q/1  "q_before"
  q/1 -> MATLAB Function/1(q)  "q_after"
  MATLAB Function/2(r1) -> reset1/1
  reset1/1 -> Integrator t1/2  "reset_after"
  x/1 -> Scope/8, MATLAB Function/2(x)
  con2/1 -> Integrator t2/1
  Integrator t1/1 -> MATLAB Function/3(y1), Scope/2  "integrator t1"
  Integrator t2/1 -> MATLAB Function/4(y2), Scope/3  "integrator t2"
  reset2/1 -> Integrator t2/2
  MATLAB Function/3(r2) -> reset2/1

== system nuclearReactor/Controller28 ==
  x : Inport
  INIT y1 : Constant  Value=0
  INIT y2 : Constant  Value=0
  Integrator t1 : DiscreteIntegrator  ExternalReset=either  InitialConditionSource=external  InitialCondition=510  InitialConditionSetting=State (most efficient)  SampleTime=-1
  Integrator t2 : DiscreteIntegrator  ExternalReset=either  InitialConditionSource=external  InitialCondition=510  InitialConditionSetting=State (most efficient)  SampleTime=-1
  MATLAB Function : MATLAB Function  Priority=1  TreatAsAtomicUnit=on
  Scope : Scope  NumInputPorts=8
      settings: TickLabels=on  ShowLegends=on  YMin=0~0~0~0~0~0~0~0  YMax=1~1~1~1~1~1~1~1
  con1 : Constant
  con2 : Constant
  q : Memory  LinearizeMemory=on
  reset1 : Memory  LinearizeMemory=on
  reset2 : Memory  LinearizeMemory=on
  control : Outport
  wires:
  MATLAB Function/4(control) -> Scope/1, control/1  "control"
  INIT y1/1 -> Integrator t1/3
  INIT y2/1 -> Integrator t2/3
  con1/1 -> Integrator t1/1
  MATLAB Function/1(qNext) -> q/1  "q_before"
  q/1 -> MATLAB Function/1(q)  "q_after"
  MATLAB Function/2(r1) -> reset1/1
  reset1/1 -> Integrator t1/2  "reset_after"
  x/1 -> Scope/8, MATLAB Function/2(x)
  con2/1 -> Integrator t2/1
  Integrator t1/1 -> MATLAB Function/3(y1), Scope/2  "integrator t1"
  Integrator t2/1 -> MATLAB Function/4(y2), Scope/3  "integrator t2"
  reset2/1 -> Integrator t2/2
  MATLAB Function/3(r2) -> reset2/1

== system nuclearReactor/Controller29 ==
  x : Inport
  INIT y1 : Constant  Value=0
  INIT y2 : Constant  Value=0
  Integrator t1 : DiscreteIntegrator  ExternalReset=either  InitialConditionSource=external  InitialCondition=510  InitialConditionSetting=State (most efficient)  SampleTime=-1
  Integrator t2 : DiscreteIntegrator  ExternalReset=either  InitialConditionSource=external  InitialCondition=510  InitialConditionSetting=State (most efficient)  SampleTime=-1
  MATLAB Function : MATLAB Function  Priority=1  TreatAsAtomicUnit=on
  Scope : Scope  NumInputPorts=8
      settings: TickLabels=on  ShowLegends=on  YMin=0~0~0~0~0~0~0~0  YMax=1~1~1~1~1~1~1~1
  con1 : Constant
  con2 : Constant
  q : Memory  LinearizeMemory=on
  reset1 : Memory  LinearizeMemory=on
  reset2 : Memory  LinearizeMemory=on
  control : Outport
  wires:
  MATLAB Function/4(control) -> Scope/1, control/1  "control"
  INIT y1/1 -> Integrator t1/3
  INIT y2/1 -> Integrator t2/3
  con1/1 -> Integrator t1/1
  MATLAB Function/1(qNext) -> q/1  "q_before"
  q/1 -> MATLAB Function/1(q)  "q_after"
  MATLAB Function/2(r1) -> reset1/1
  reset1/1 -> Integrator t1/2  "reset_after"
  x/1 -> Scope/8, MATLAB Function/2(x)
  con2/1 -> Integrator t2/1
  Integrator t1/1 -> MATLAB Function/3(y1), Scope/2  "integrator t1"
  Integrator t2/1 -> MATLAB Function/4(y2), Scope/3  "integrator t2"
  reset2/1 -> Integrator t2/2
  MATLAB Function/3(r2) -> reset2/1

== system nuclearReactor/Controller3 ==
  x : Inport
  INIT y1 : Constant  Value=0
  INIT y2 : Constant  Value=0
  Integrator t1 : DiscreteIntegrator  ExternalReset=either  InitialConditionSource=external  InitialCondition=510  InitialConditionSetting=State (most efficient)  SampleTime=-1
  Integrator t2 : DiscreteIntegrator  ExternalReset=either  InitialConditionSource=external  InitialCondition=510  InitialConditionSetting=State (most efficient)  SampleTime=-1
  MATLAB Function : MATLAB Function  Priority=1  TreatAsAtomicUnit=on
  Scope : Scope  NumInputPorts=8
      settings: TickLabels=on  ShowLegends=on  YMin=0~0~0~0~0~0~0~0  YMax=1~1~1~1~1~1~1~1
  con1 : Constant
  con2 : Constant
  q : Memory  LinearizeMemory=on
  reset1 : Memory  LinearizeMemory=on
  reset2 : Memory  LinearizeMemory=on
  control : Outport
  wires:
  MATLAB Function/4(control) -> Scope/1, control/1  "control"
  INIT y1/1 -> Integrator t1/3
  INIT y2/1 -> Integrator t2/3
  con1/1 -> Integrator t1/1
  MATLAB Function/1(qNext) -> q/1  "q_before"
  q/1 -> MATLAB Function/1(q)  "q_after"
  MATLAB Function/2(r1) -> reset1/1
  reset1/1 -> Integrator t1/2  "reset_after"
  x/1 -> Scope/8, MATLAB Function/2(x)
  con2/1 -> Integrator t2/1
  Integrator t1/1 -> MATLAB Function/3(y1), Scope/2  "integrator t1"
  Integrator t2/1 -> MATLAB Function/4(y2), Scope/3  "integrator t2"
  reset2/1 -> Integrator t2/2
  MATLAB Function/3(r2) -> reset2/1

== system nuclearReactor/Controller4 ==
  x : Inport
  INIT y1 : Constant  Value=0
  INIT y2 : Constant  Value=0
  Integrator t1 : DiscreteIntegrator  ExternalReset=either  InitialConditionSource=external  InitialCondition=510  InitialConditionSetting=State (most efficient)  SampleTime=-1
  Integrator t2 : DiscreteIntegrator  ExternalReset=either  InitialConditionSource=external  InitialCondition=510  InitialConditionSetting=State (most efficient)  SampleTime=-1
  MATLAB Function : MATLAB Function  Priority=1  TreatAsAtomicUnit=on
  Scope : Scope  NumInputPorts=8
      settings: TickLabels=on  ShowLegends=on  YMin=0~0~0~0~0~0~0~0  YMax=1~1~1~1~1~1~1~1
  con1 : Constant
  con2 : Constant
  q : Memory  LinearizeMemory=on
  reset1 : Memory  LinearizeMemory=on
  reset2 : Memory  LinearizeMemory=on
  control : Outport
  wires:
  MATLAB Function/4(control) -> Scope/1, control/1  "control"
  INIT y1/1 -> Integrator t1/3
  INIT y2/1 -> Integrator t2/3
  con1/1 -> Integrator t1/1
  MATLAB Function/1(qNext) -> q/1  "q_before"
  q/1 -> MATLAB Function/1(q)  "q_after"
  MATLAB Function/2(r1) -> reset1/1
  reset1/1 -> Integrator t1/2  "reset_after"
  x/1 -> Scope/8, MATLAB Function/2(x)
  con2/1 -> Integrator t2/1
  Integrator t1/1 -> MATLAB Function/3(y1), Scope/2  "integrator t1"
  Integrator t2/1 -> MATLAB Function/4(y2), Scope/3  "integrator t2"
  reset2/1 -> Integrator t2/2
  MATLAB Function/3(r2) -> reset2/1

== system nuclearReactor/Controller5 ==
  x : Inport
  INIT y1 : Constant  Value=0
  INIT y2 : Constant  Value=0
  Integrator t1 : DiscreteIntegrator  ExternalReset=either  InitialConditionSource=external  InitialCondition=510  InitialConditionSetting=State (most efficient)  SampleTime=-1
  Integrator t2 : DiscreteIntegrator  ExternalReset=either  InitialConditionSource=external  InitialCondition=510  InitialConditionSetting=State (most efficient)  SampleTime=-1
  MATLAB Function : MATLAB Function  Priority=1  TreatAsAtomicUnit=on
  Scope : Scope  NumInputPorts=8
      settings: TickLabels=on  ShowLegends=on  YMin=0~0~0~0~0~0~0~0  YMax=1~1~1~1~1~1~1~1
  con1 : Constant
  con2 : Constant
  q : Memory  LinearizeMemory=on
  reset1 : Memory  LinearizeMemory=on
  reset2 : Memory  LinearizeMemory=on
  control : Outport
  wires:
  MATLAB Function/4(control) -> Scope/1, control/1  "control"
  INIT y1/1 -> Integrator t1/3
  INIT y2/1 -> Integrator t2/3
  con1/1 -> Integrator t1/1
  MATLAB Function/1(qNext) -> q/1  "q_before"
  q/1 -> MATLAB Function/1(q)  "q_after"
  MATLAB Function/2(r1) -> reset1/1
  reset1/1 -> Integrator t1/2  "reset_after"
  x/1 -> Scope/8, MATLAB Function/2(x)
  con2/1 -> Integrator t2/1
  Integrator t1/1 -> MATLAB Function/3(y1), Scope/2  "integrator t1"
  Integrator t2/1 -> MATLAB Function/4(y2), Scope/3  "integrator t2"
  reset2/1 -> Integrator t2/2
  MATLAB Function/3(r2) -> reset2/1

== system nuclearReactor/Controller6 ==
  x : Inport
  INIT y1 : Constant  Value=0
  INIT y2 : Constant  Value=0
  Integrator t1 : DiscreteIntegrator  ExternalReset=either  InitialConditionSource=external  InitialCondition=510  InitialConditionSetting=State (most efficient)  SampleTime=-1
  Integrator t2 : DiscreteIntegrator  ExternalReset=either  InitialConditionSource=external  InitialCondition=510  InitialConditionSetting=State (most efficient)  SampleTime=-1
  MATLAB Function : MATLAB Function  Priority=1  TreatAsAtomicUnit=on
  Scope : Scope  NumInputPorts=8
      settings: TickLabels=on  ShowLegends=on  YMin=0~0~0~0~0~0~0~0  YMax=1~1~1~1~1~1~1~1
  con1 : Constant
  con2 : Constant
  q : Memory  LinearizeMemory=on
  reset1 : Memory  LinearizeMemory=on
  reset2 : Memory  LinearizeMemory=on
  control : Outport
  wires:
  MATLAB Function/4(control) -> Scope/1, control/1  "control"
  INIT y1/1 -> Integrator t1/3
  INIT y2/1 -> Integrator t2/3
  con1/1 -> Integrator t1/1
  MATLAB Function/1(qNext) -> q/1  "q_before"
  q/1 -> MATLAB Function/1(q)  "q_after"
  MATLAB Function/2(r1) -> reset1/1
  reset1/1 -> Integrator t1/2  "reset_after"
  x/1 -> Scope/8, MATLAB Function/2(x)
  con2/1 -> Integrator t2/1
  Integrator t1/1 -> MATLAB Function/3(y1), Scope/2  "integrator t1"
  Integrator t2/1 -> MATLAB Function/4(y2), Scope/3  "integrator t2"
  reset2/1 -> Integrator t2/2
  MATLAB Function/3(r2) -> reset2/1

== system nuclearReactor/Controller7 ==
  x : Inport
  INIT y1 : Constant  Value=0
  INIT y2 : Constant  Value=0
  Integrator t1 : DiscreteIntegrator  ExternalReset=either  InitialConditionSource=external  InitialCondition=510  InitialConditionSetting=State (most efficient)  SampleTime=-1
  Integrator t2 : DiscreteIntegrator  ExternalReset=either  InitialConditionSource=external  InitialCondition=510  InitialConditionSetting=State (most efficient)  SampleTime=-1
  MATLAB Function : MATLAB Function  Priority=1  TreatAsAtomicUnit=on
  Scope : Scope  NumInputPorts=8
      settings: TickLabels=on  ShowLegends=on  YMin=0~0~0~0~0~0~0~0  YMax=1~1~1~1~1~1~1~1
  con1 : Constant
  con2 : Constant
  q : Memory  LinearizeMemory=on
  reset1 : Memory  LinearizeMemory=on
  reset2 : Memory  LinearizeMemory=on
  control : Outport
  wires:
  MATLAB Function/4(control) -> Scope/1, control/1  "control"
  INIT y1/1 -> Integrator t1/3
  INIT y2/1 -> Integrator t2/3
  con1/1 -> Integrator t1/1
  MATLAB Function/1(qNext) -> q/1  "q_before"
  q/1 -> MATLAB Function/1(q)  "q_after"
  MATLAB Function/2(r1) -> reset1/1
  reset1/1 -> Integrator t1/2  "reset_after"
  x/1 -> Scope/8, MATLAB Function/2(x)
  con2/1 -> Integrator t2/1
  Integrator t1/1 -> MATLAB Function/3(y1), Scope/2  "integrator t1"
  Integrator t2/1 -> MATLAB Function/4(y2), Scope/3  "integrator t2"
  reset2/1 -> Integrator t2/2
  MATLAB Function/3(r2) -> reset2/1

== system nuclearReactor/Controller8 ==
  x : Inport
  INIT y1 : Constant  Value=0
  INIT y2 : Constant  Value=0
  Integrator t1 : DiscreteIntegrator  ExternalReset=either  InitialConditionSource=external  InitialCondition=510  InitialConditionSetting=State (most efficient)  SampleTime=-1
  Integrator t2 : DiscreteIntegrator  ExternalReset=either  InitialConditionSource=external  InitialCondition=510  InitialConditionSetting=State (most efficient)  SampleTime=-1
  MATLAB Function : MATLAB Function  Priority=1  TreatAsAtomicUnit=on
  Scope : Scope  NumInputPorts=8
      settings: TickLabels=on  ShowLegends=on  YMin=0~0~0~0~0~0~0~0  YMax=1~1~1~1~1~1~1~1
  con1 : Constant
  con2 : Constant
  q : Memory  LinearizeMemory=on
  reset1 : Memory  LinearizeMemory=on
  reset2 : Memory  LinearizeMemory=on
  control : Outport
  wires:
  MATLAB Function/4(control) -> Scope/1, control/1  "control"
  INIT y1/1 -> Integrator t1/3
  INIT y2/1 -> Integrator t2/3
  con1/1 -> Integrator t1/1
  MATLAB Function/1(qNext) -> q/1  "q_before"
  q/1 -> MATLAB Function/1(q)  "q_after"
  MATLAB Function/2(r1) -> reset1/1
  reset1/1 -> Integrator t1/2  "reset_after"
  x/1 -> Scope/8, MATLAB Function/2(x)
  con2/1 -> Integrator t2/1
  Integrator t1/1 -> MATLAB Function/3(y1), Scope/2  "integrator t1"
  Integrator t2/1 -> MATLAB Function/4(y2), Scope/3  "integrator t2"
  reset2/1 -> Integrator t2/2
  MATLAB Function/3(r2) -> reset2/1

== system nuclearReactor/Controller9 ==
  x : Inport
  INIT y1 : Constant  Value=0
  INIT y2 : Constant  Value=0
  Integrator t1 : DiscreteIntegrator  ExternalReset=either  InitialConditionSource=external  InitialCondition=510  InitialConditionSetting=State (most efficient)  SampleTime=-1
  Integrator t2 : DiscreteIntegrator  ExternalReset=either  InitialConditionSource=external  InitialCondition=510  InitialConditionSetting=State (most efficient)  SampleTime=-1
  MATLAB Function : MATLAB Function  Priority=1  TreatAsAtomicUnit=on
  Scope : Scope  NumInputPorts=8
      settings: TickLabels=on  ShowLegends=on  YMin=0~0~0~0~0~0~0~0  YMax=1~1~1~1~1~1~1~1
  con1 : Constant
  con2 : Constant
  q : Memory  LinearizeMemory=on
  reset1 : Memory  LinearizeMemory=on
  reset2 : Memory  LinearizeMemory=on
  control : Outport
  wires:
  MATLAB Function/4(control) -> Scope/1, control/1  "control"
  INIT y1/1 -> Integrator t1/3
  INIT y2/1 -> Integrator t2/3
  con1/1 -> Integrator t1/1
  MATLAB Function/1(qNext) -> q/1  "q_before"
  q/1 -> MATLAB Function/1(q)  "q_after"
  MATLAB Function/2(r1) -> reset1/1
  reset1/1 -> Integrator t1/2  "reset_after"
  x/1 -> Scope/8, MATLAB Function/2(x)
  con2/1 -> Integrator t2/1
  Integrator t1/1 -> MATLAB Function/3(y1), Scope/2  "integrator t1"
  Integrator t2/1 -> MATLAB Function/4(y2), Scope/3  "integrator t2"
  reset2/1 -> Integrator t2/2
  MATLAB Function/3(r2) -> reset2/1
